simulink model "TST_EngPrt_TrqLimPTO"  (R2016b)
settings: Solver=FixedStepDiscrete  StartTime=0.0  StopTime=simTime  FixedStep=sampleTime  RelTol=1e-3
values from neighbouring files (symbols this model uses):
  testCase = 1    [initTST_EngPrt_TrqLimPTO_001.m]
libraries: simulink x3, UnitTest_Lib x1
settings Model: Creator=zhengjinyan  LastModifiedBy=zhengjinyan
settings DebuggingCC: SignalRangeChecking=error

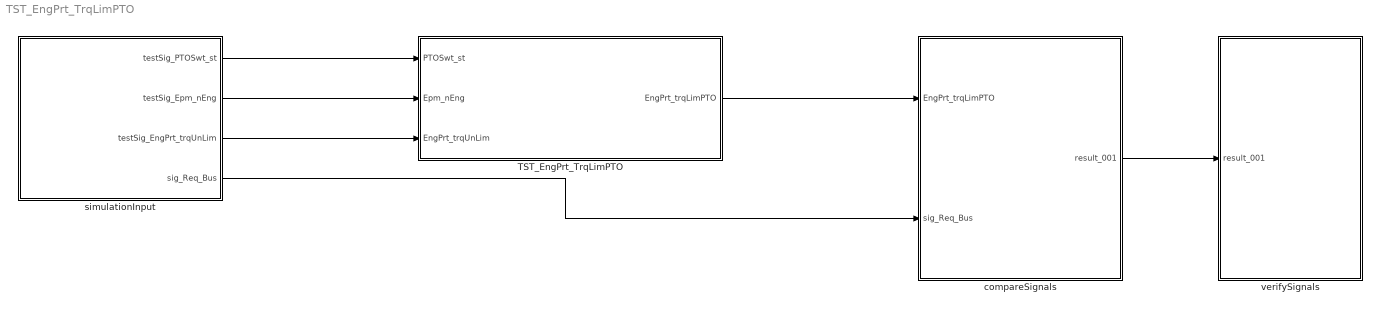
== system TST_EngPrt_TrqLimPTO ==
  TST_EngPrt_TrqLimPTO : Subsystem
  compareSignals : Subsystem
  simulationInput : Subsystem
  verifySignals : Subsystem
  wires:
  simulationInput/1(testSig_PTOSwt_st) -> TST_EngPrt_TrqLimPTO/1(PTOSwt_st)
  simulationInput/2(testSig_Epm_nEng) -> TST_EngPrt_TrqLimPTO/2(Epm_nEng)
  simulationInput/3(testSig_EngPrt_trqUnLim) -> TST_EngPrt_TrqLimPTO/3(EngPrt_trqUnLim)
  TST_EngPrt_TrqLimPTO/1(EngPrt_trqLimPTO) -> compareSignals/1(EngPrt_trqLimPTO)
  simulationInput/4(sig_Req_Bus) -> compareSignals/2(sig_Req_Bus)
  compareSignals/1(result_001) -> verifySignals/1(result_001)

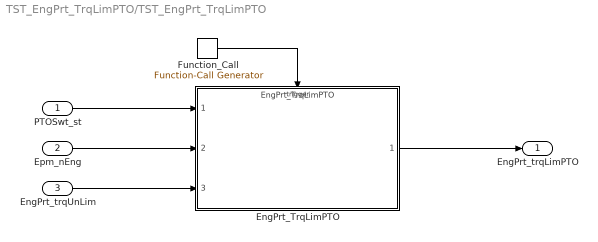
== system TST_EngPrt_TrqLimPTO/TST_EngPrt_TrqLimPTO ==
  PTOSwt_st : Inport
  Epm_nEng : Inport  Port=2
  EngPrt_trqUnLim : Inport  Port=3
  EngPrt_TrqLimPTO : ModelReference  ModelNameDialog=EngPrt_TrqLimPTO  SimulationMode=Normal  ModelReferenceVersion=1.11  TriggerPortName=function  TriggerPortTriggerType=function-call  TriggerPortStatesWhenEnabling=held
  Function_Call : simulink/Ports & Subsystems/Function-Call Generator  sample_time=sampleTime  numberOfIterations=1
  EngPrt_trqLimPTO : Outport
  wires:
  Function_Call/1 -> EngPrt_TrqLimPTO/Trigger
  PTOSwt_st/1 -> EngPrt_TrqLimPTO/1
  Epm_nEng/1 -> EngPrt_TrqLimPTO/2
  EngPrt_trqUnLim/1 -> EngPrt_TrqLimPTO/3
  EngPrt_TrqLimPTO/1 -> EngPrt_trqLimPTO/1

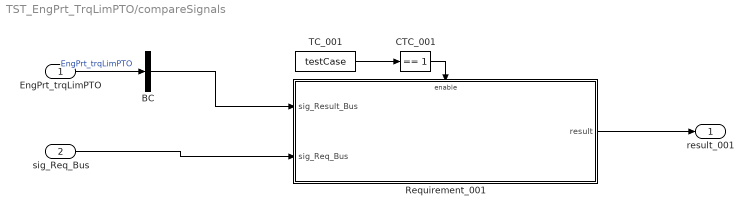
== system TST_EngPrt_TrqLimPTO/compareSignals ==
  EngPrt_trqLimPTO : Inport
  sig_Req_Bus : Inport  Port=2
  BC : BusCreator  Inputs=1
  CTC_001 : simulink/Logic and Bit Operations/Compare To Constant  relop===  const=1  OutDataTypeStr=boolean
  Requirement_001 : Subsystem
  TC_001 : Constant  Value=testCase
  result_001 : Outport
  wires:
  EngPrt_trqLimPTO/1 -> BC/1  "EngPrt_trqLimPTO"
  TC_001/1 -> CTC_001/1
  CTC_001/1 -> Requirement_001/Enable
  sig_Req_Bus/1 -> Requirement_001/2(sig_Req_Bus)
  BC/1 -> Requirement_001/1(sig_Result_Bus)
  Requirement_001/1(result) -> result_001/1

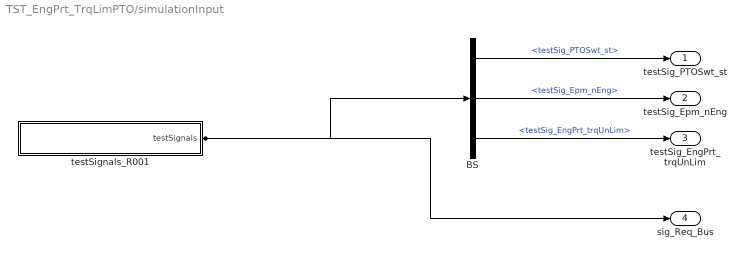
== system TST_EngPrt_TrqLimPTO/simulationInput ==
  BS : BusSelector  OutputSignals=testSig_PTOSwt_st,testSig_Epm_nEng,testSig_EngPrt_trqUnLim
  testSignals_R001 : Subsystem
  testSig_PTOSwt_st : Outport
  testSig_Epm_nEng : Outport  Port=2
  testSig_EngPrt_trqUnLim : Outport  Port=3
  sig_Req_Bus : Outport  Port=4
  wires:
  BS/1 -> testSig_PTOSwt_st/1  "<testSig_PTOSwt_st>"
  BS/2 -> testSig_Epm_nEng/1  "<testSig_Epm_nEng>"
  BS/3 -> testSig_EngPrt_trqUnLim/1  "<testSig_EngPrt_trqUnLim>"
  testSignals_R001/1(testSignals) -> BS/1, sig_Req_Bus/1

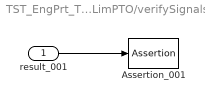
== system TST_EngPrt_TrqLimPTO/verifySignals ==
  result_001 : Inport
  Assertion_001 : Assertion  Enabled=off
  wires:
  result_001/1 -> Assertion_001/1

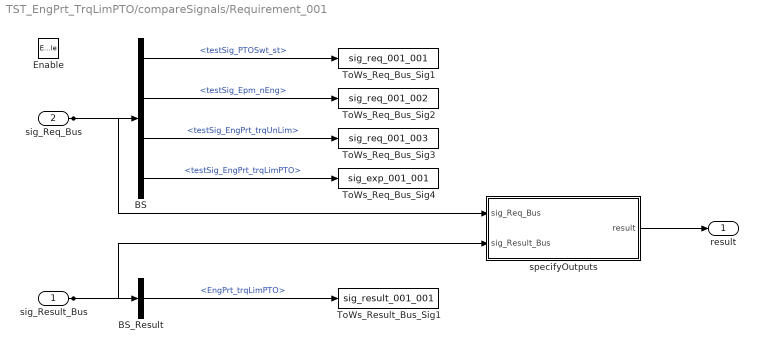
== system TST_EngPrt_TrqLimPTO/compareSignals/Requirement_001 ==
  sig_Result_Bus : Inport
  sig_Req_Bus : Inport  Port=2
  Enable : EnablePort
  BS : BusSelector  OutputSignals=testSig_PTOSwt_st,testSig_Epm_nEng,testSig_EngPrt_trqUnLim,testSig_EngPrt_trqLimPTO
  BS_Result : BusSelector  OutputSignals=EngPrt_trqLimPTO
  ToWs_Req_Bus_Sig1 : ToWorkspace  VariableName=sig_req_001_001  SaveFormat=Structure With Time
  ToWs_Req_Bus_Sig2 : ToWorkspace  VariableName=sig_req_001_002  SaveFormat=Structure With Time
  ToWs_Req_Bus_Sig3 : ToWorkspace  VariableName=sig_req_001_003  SaveFormat=Structure With Time
  ToWs_Req_Bus_Sig4 : ToWorkspace  VariableName=sig_exp_001_001  SaveFormat=Structure With Time
  ToWs_Result_Bus_Sig1 : ToWorkspace  VariableName=sig_result_001_001  SaveFormat=Structure With Time
  specifyOutputs : Subsystem
  result : Outport
  wires:
  sig_Req_Bus/1 -> BS/1, specifyOutputs/1(sig_Req_Bus)
  BS/1 -> ToWs_Req_Bus_Sig1/1  "<testSig_PTOSwt_st>"
  BS/2 -> ToWs_Req_Bus_Sig2/1  "<testSig_Epm_nEng>"
  BS/3 -> ToWs_Req_Bus_Sig3/1  "<testSig_EngPrt_trqUnLim>"
  BS/4 -> ToWs_Req_Bus_Sig4/1  "<testSig_EngPrt_trqLimPTO>"
  sig_Result_Bus/1 -> BS_Result/1, specifyOutputs/2(sig_Result_Bus)
  BS_Result/1 -> ToWs_Result_Bus_Sig1/1  "<EngPrt_trqLimPTO>"
  specifyOutputs/1(result) -> result/1

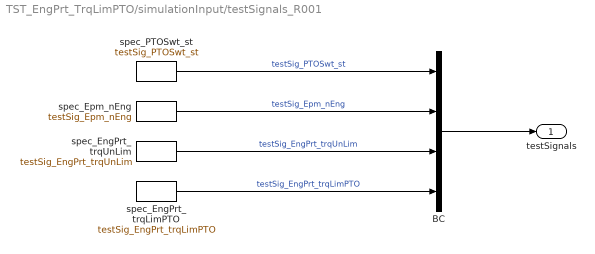
== system TST_EngPrt_TrqLimPTO/simulationInput/testSignals_R001 ==
  BC : BusCreator  Inputs=4
  spec_EngPrt_trqLimPTO : FromWorkspace  VariableName=testSig_EngPrt_trqLimPTO  Interpolate=off  OutputAfterFinalValue=Holding final value
  spec_EngPrt_trqUnLim : FromWorkspace  VariableName=testSig_EngPrt_trqUnLim  Interpolate=off  OutputAfterFinalValue=Holding final value
  spec_Epm_nEng : FromWorkspace  VariableName=testSig_Epm_nEng  Interpolate=off  OutputAfterFinalValue=Holding final value
  spec_PTOSwt_st : FromWorkspace  VariableName=testSig_PTOSwt_st  Interpolate=off  OutputAfterFinalValue=Holding final value
  testSignals : Outport
  wires:
  BC/1 -> testSignals/1
  spec_PTOSwt_st/1 -> BC/1  "testSig_PTOSwt_st"
  spec_Epm_nEng/1 -> BC/2  "testSig_Epm_nEng"
  spec_EngPrt_trqUnLim/1 -> BC/3  "testSig_EngPrt_trqUnLim"
  spec_EngPrt_trqLimPTO/1 -> BC/4  "testSig_EngPrt_trqLimPTO"

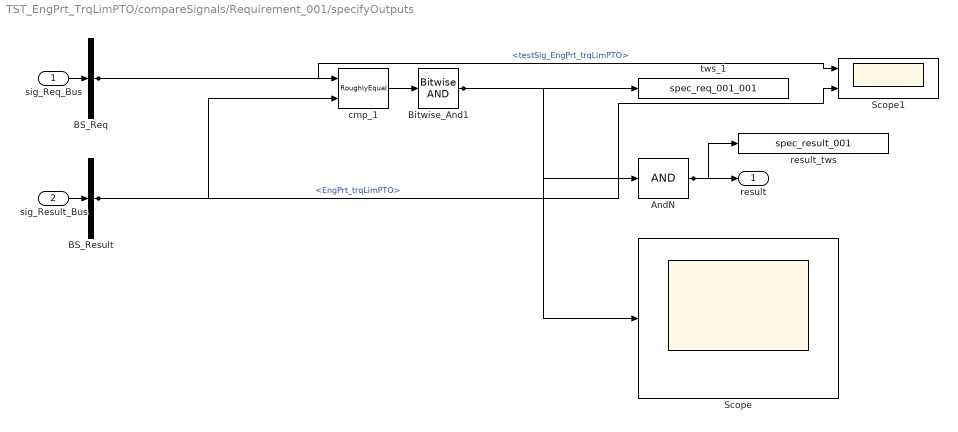
== system TST_EngPrt_TrqLimPTO/compareSignals/Requirement_001/specifyOutputs ==
  sig_Req_Bus : Inport
  sig_Result_Bus : Inport  Port=2
  AndN : Logic  Inputs=1
  BS_Req : BusSelector  OutputSignals=testSig_EngPrt_trqLimPTO
  BS_Result : BusSelector  OutputSignals=EngPrt_trqLimPTO
  Bitwise_And1 : simulink/Logic and Bit Operations/Bitwise Operator  logicop=AND  UseBitMask=off  BitMask=bin2dec('11011001')  BitMaskRealWorld=Stored Integer
  Scope : Scope
  Scope1 : Scope  NumInputPorts=2
  cmp_1 : UnitTest_Lib/RoughlyEqual  slope=0.1
  result_tws : ToWorkspace  VariableName=spec_result_001
  tws_1 : ToWorkspace  VariableName=spec_req_001_001
  result : Outport
  wires:
  sig_Req_Bus/1 -> BS_Req/1
  sig_Result_Bus/1 -> BS_Result/1
  AndN/1 -> result/1, result_tws/1
  BS_Req/1 -> cmp_1/1, Scope1/1  "<testSig_EngPrt_trqLimPTO>"
  BS_Result/1 -> cmp_1/2, Scope1/2  "<EngPrt_trqLimPTO>"
  cmp_1/1 -> Bitwise_And1/1
  Bitwise_And1/1 -> tws_1/1, AndN/1, Scope/1
